simulink model "MEGA2560hex_OneWire_task"  (Simulink 7.0)
libraries: logiclib x10, REXduino_library x9, mathlib x6, arclib x2, genlib x1
settings Model: Creator=Jarda  LastModifiedBy=Jarda  ExtModeTrigMode=oneshot  ExtModeArmWhenConnect=off

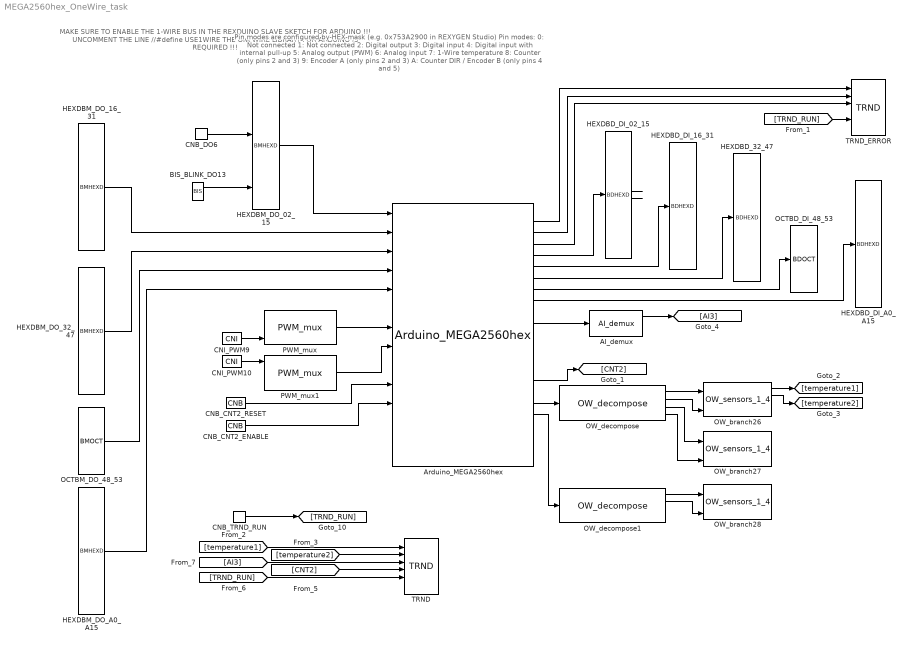
== system MEGA2560hex_OneWire_task ==
  note: MAKE SURE TO ENABLE THE 1-WIRE BUS IN
      | THE REXDUINO SLAVE SKETCH FOR ARDUINO !!!
      |
      | UNCOMMENT THE LINE //#define USE1WIRE
      | THE ONEWIRE LIBRARY FOR ARDUINO IS REQUIRED !!!
  note: Pin modes are configured by HEX mask
      |    (e.g. 0x753A2900 in REXYGEN Studio)
      |
      | Pin modes:
      | 0: Not connected
      | 1: Not connected
      | 2: Digital output
      | 3: Digital input
      | 4: Digital input with internal pull-up
      | 5: Analog output (PWM)
      | 6: Analog input
      | 7: 1-Wire temperature
      | 8: Counter (only pins 2 and 3)
      | 9: Encoder A (only pins 2 and 3)
      | A: Counter DIR / Encoder B (only pins 4 and 5)
  AI_demux : REXduino_library/AI_demux
      mask Type: REX sequence
  Arduino_MEGA2560hex : REXduino_library/Arduino_MEGA2560hex  comPort=/dev/ttyACM0  pinmodes_00_07=0x320A0800  pinmodes_08_15=0x00200554  pinmodes_16_23=0  pinmodes_24_31=0x00077700  pinmodes_32_39=0  pinmodes_40_47=0  pinmodes_48_53=0  pinmodes_A0_A7=0x00006000  pinmodes_A8_A15=0  usercmd=1: No data
  BIS_BLINK_DO13 : genlib/BIS  Y0=off  t1=2  t2=4  t3=0  t4=4  t5=5  t6=6  t7=7  t8=8  RPT=on
  CNB_CNT2_ENABLE : mathlib/CNB  YCN=on
  CNB_CNT2_RESET : mathlib/CNB  YCN=off
  CNB_DO6 : mathlib/CNB  YCN=on
  CNB_TRND_RUN : mathlib/CNB  YCN=on
  CNI_PWM10 : mathlib/CNI  icn=128
  CNI_PWM9 : mathlib/CNI  icn=128
  HEXDBD_32_47 : logiclib/BDHEXD  shift=0
  HEXDBD_DI_02_15 : logiclib/BDHEXD  shift=0
  HEXDBD_DI_16_31 : logiclib/BDHEXD  shift=0
  HEXDBD_DI_A0_A15 : logiclib/BDHEXD  shift=0
  HEXDBM_DO_02_15 : logiclib/BMHEXD  shift=0
  HEXDBM_DO_16_31 : logiclib/BMHEXD  shift=0
  HEXDBM_DO_32_47 : logiclib/BMHEXD  shift=0
  HEXDBM_DO_A0_A15 : logiclib/BMHEXD  shift=0
  OCTBD_DI_48_53 : logiclib/BDOCT  shift=0
  OCTBM_DO_48_53 : logiclib/BMOCT  shift=0
  OW_branch26 : REXduino_library/OW_sensors_1_4
      mask Type: REX sequence
  OW_branch27 : REXduino_library/OW_sensors_1_4
      mask Type: REX sequence
  OW_branch28 : REXduino_library/OW_sensors_1_4
      mask Type: REX sequence
  OW_decompose : REXduino_library/OW_decompose
      mask Type: REX sequence
  OW_decompose1 : REXduino_library/OW_decompose
      mask Type: REX sequence
  PWM_mux : REXduino_library/PWM_mux
      mask Type: REX sequence
  PWM_mux1 : REXduino_library/PWM_mux
      mask Type: REX sequence
  TRND : arclib/TRND  n=4  l=14400  btype=8: Double  ptype1=1: Store  ptype2=1: Store  ptype3=1: Store  ptype4=1: Store  pfac=1  afac=0  arc=0  id=1  Title=Data trend  timesrc=1
  TRND_ERROR : arclib/TRND  n=4  l=1000  btype=8: Double  ptype1=1: Store  ptype2=1: Store  ptype3=1: Store  ptype4=1: Store  pfac=1  afac=0  arc=0  id=1  Title=ERROR trend  timesrc=1
  wires:
  AI_demux/1 -> [AI3]
  Arduino_MEGA2560hex/1 -> TRND_ERROR/1
  Arduino_MEGA2560hex/2 -> TRND_ERROR/2
  Arduino_MEGA2560hex/3 -> TRND_ERROR/3
  Arduino_MEGA2560hex/4 -> HEXDBD_DI_02_15/1
  Arduino_MEGA2560hex/5 -> HEXDBD_DI_16_31/1
  Arduino_MEGA2560hex/6 -> HEXDBD_32_47/1
  Arduino_MEGA2560hex/7 -> OCTBD_DI_48_53/1
  Arduino_MEGA2560hex/8 -> HEXDBD_DI_A0_A15/1
  Arduino_MEGA2560hex/10 -> AI_demux/1
  Arduino_MEGA2560hex/15 -> [CNT2]
  Arduino_MEGA2560hex/17 -> OW_decompose/1
  Arduino_MEGA2560hex/18 -> OW_decompose1/1
  BIS_BLINK_DO13/1 -> HEXDBM_DO_02_15/14
  CNB_CNT2_ENABLE/1 -> Arduino_MEGA2560hex/11
  CNB_CNT2_RESET/1 -> Arduino_MEGA2560hex/10
  CNB_DO6/1 -> HEXDBM_DO_02_15/7
  CNB_TRND_RUN/1 -> [TRND_RUN]
  CNI_PWM10/1 -> PWM_mux1/1
  CNI_PWM9/1 -> PWM_mux/4
  [TRND_RUN] -> TRND_ERROR/5
  [temperature1] -> TRND/1
  [temperature2] -> TRND/2
  [CNT2] -> TRND/4
  [TRND_RUN] -> TRND/5
  [AI3] -> TRND/3
  HEXDBD_DI_02_15/8 -> ?
  HEXDBD_DI_02_15/9 -> ?
  HEXDBM_DO_02_15/1 -> Arduino_MEGA2560hex/1
  HEXDBM_DO_16_31/1 -> Arduino_MEGA2560hex/2
  HEXDBM_DO_32_47/1 -> Arduino_MEGA2560hex/3
  HEXDBM_DO_A0_A15/1 -> Arduino_MEGA2560hex/5
  OCTBM_DO_48_53/1 -> Arduino_MEGA2560hex/4
  OW_branch26/1 -> [temperature1]
  OW_branch26/2 -> [temperature2]
  OW_decompose/1 -> OW_branch26/1
  OW_decompose/2 -> OW_branch26/2
  OW_decompose/3 -> OW_branch27/1
  OW_decompose/4 -> OW_branch27/2
  OW_decompose1/1 -> OW_branch28/1
  OW_decompose1/2 -> OW_branch28/2
  PWM_mux/1 -> Arduino_MEGA2560hex/7
  PWM_mux1/1 -> Arduino_MEGA2560hex/8
